simulink model "h08_numpy_matlab_simulink"  (R2026a)
settings: Solver=VariableStepAuto
values from neighbouring files (symbols this model uses):
  A = [0  1; -1  -0.5]    [e05_matlab_export.mat]    (also in e05_python_export.mat = [1  2  3; 4  5  6]; statesapce_data.mat; statespace_data.mat)
  B = [0 1]    [statesapce_data.mat]    (also in statespace_data.mat)
  C = [1  0; 0  1]    [statesapce_data.mat]    (also in statespace_data.mat)
  D = [0 0]    [statesapce_data.mat]    (also in statespace_data.mat)
settings Model: Creator=itsyu  LastModifiedBy=itsyu

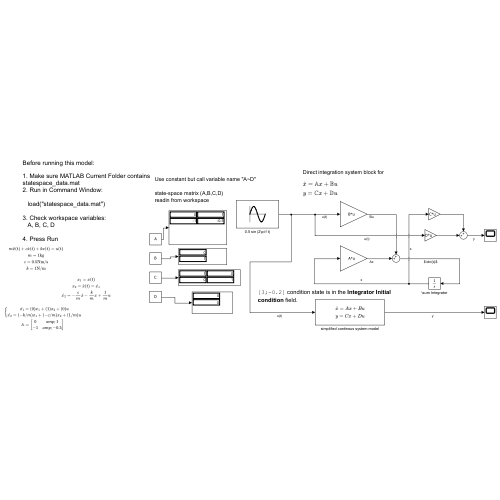
[thumbnail: Simulink's stored preview of the top-level diagram]
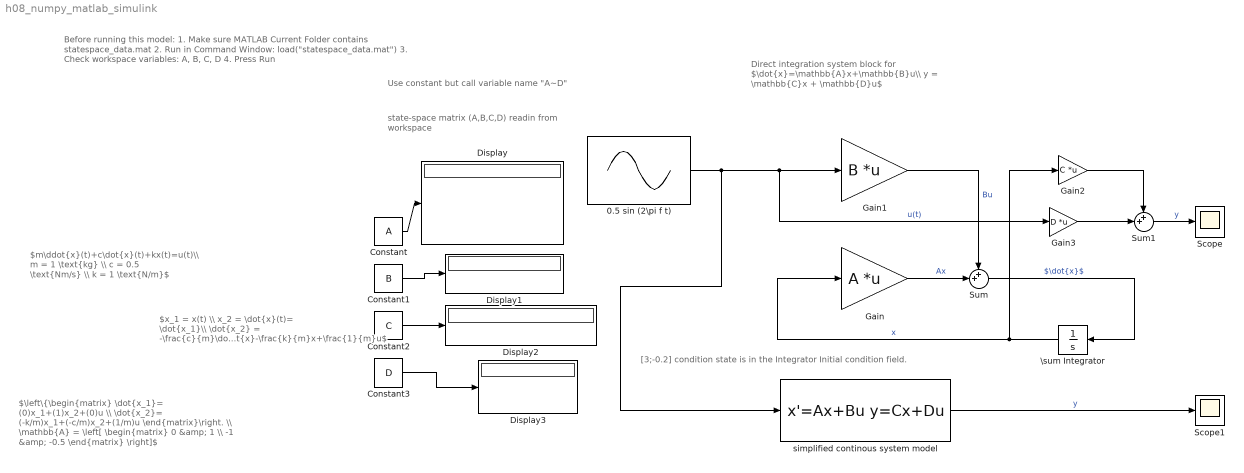
== system h08_numpy_matlab_simulink ==
  note: $m\ddot{x}(t)+c\dot{x}(t)+kx(t)=u(t)\\ m = 1 \text{kg} \\ c = 0.5 \text{Nm/s} \\ k = 1 \text{N/m}$
  note: Use constant but call variable name "A~D"
  note: [3;-0.2] condition state is in the Integrator Initial condition field.
  note: state-space matrix (A,B,C,D)
      | readin from workspace
  note: Before running this model:
      |
      | 1. Make sure MATLAB Current Folder contains statespace_data.mat
      | 2. Run in Command Window:
      |
      | load("statespace_data.mat")
      |
      | 3. Check workspace variables:
      | A, B, C, D
      |
      | 4. Press Run
  note: Direct integration system block for
      |
      | $\dot{x}=\mathbb{A}x+\mathbb{B}u\\ y = \mathbb{C}x + \mathbb{D}u$
  note: $x_1 = x(t) \\ x_2 = \dot{x}(t)= \dot{x_1}\\ \dot{x_2} = -\frac{c}{m}\dot{x}-\frac{k}{m}x+\frac{1}{m}u$
  note: $\left\{\begin{matrix} \dot{x_1}= (0)x_1+(1)x_2+(0)u \\ \dot{x_2}= (-k/m)x_1+(-c/m)x_2+(1/m)u \end{matrix}\right. \\ \mathbb{A} = \left[ \begin{matrix} 0 &amp; 1 \\ -1 &amp; -0.5 \end{matrix} \right]$
  0.5 sin (2\pi f t) : Sin  Amplitude=0.5  SampleTime=0
  Constant : Constant  Value=A
  Constant1 : Constant  Value=B
  Constant2 : Constant  Value=C
  Constant3 : Constant  Value=D
  Display{,1..3} (4 alike) : Display
  Gain : Gain  Gain=A  Multiplication=Matrix(K*u)
  Gain1 : Gain  Gain=B  Multiplication=Matrix(K*u)
  Gain2 : Gain  Gain=C  Multiplication=Matrix(K*u)
  Gain3 : Gain  Gain=D  Multiplication=Matrix(K*u)
  Scope : Scope
      settings: ActiveDisplayYMinimum=-2.501184627917044  ActiveDisplayYMaximum=3.6112427364352269
  Scope1 : Scope
      settings: ActiveDisplayYMinimum=-2.501184627917044  ActiveDisplayYMaximum=3.6112427364352269
  Sum : Sum  Inputs=++|
  Sum1 : Sum  Inputs=++|
  \sum Integrator : Integrator  InitialCondition=[3;-0.2]
  simplified continous system model : StateSpace  A=A  B=B  C=C  D=D  InitialCondition=[3;-0.2]
  wires:
  Constant/1 -> Display/1
  Constant1/1 -> Display1/1
  Constant2/1 -> Display2/1
  Constant3/1 -> Display3/1
  0.5 sin (2\pi f t)/1 -> simplified continous system model/1, Gain3/1, Gain1/1  "u(t)"
  Gain/1 -> Sum/2  "Ax"
  Gain1/1 -> Sum/1  "Bu"
  Sum/1 -> \sum Integrator/1  "$\\dot{x}$"
  \sum Integrator/1 -> Gain2/1, Gain/1  "x"
  Gain2/1 -> Sum1/1
  Sum1/1 -> Scope/1  "y"
  Gain3/1 -> Sum1/2
  simplified continous system model/1 -> Scope1/1  "y"
